simulink model "ResonantEstimator"  (R2019b)
settings: Solver=VariableStepAuto  StartTime=0.0  StopTime=tSim  RelTol=1e-3
values from neighbouring files (symbols this model uses):
  a = 0    [Q4.m]    (also in Sol_Q1.m = 0.1)
  amplitude = 3    [Q4.m]
  deltat = 0.01    [Q4.m]    (also in Sol_Q1.m = 0.001; main3.m; param3.m = 0.001; params2.m = 0.1)
  gamma1 = (2*zeta*wn)/b    (= 4)    [Q4.m]
  gamma2 = (wn^2 - w0^2)/b    (= 7.5)    [Q4.m]
  Gs = tf(b, [1 a])    [Q4.m]    (also in Q5.m = tf([b1 b0], [1 a1 a0]); Sol_Q1.m = tf(num, den); main3.m = tf(num, den); param3.m = tf(b, [1 a1 a0]))
  K1 = (alpha1 - a)/b    (= 1.5)    [Q4.m]    (also in Sol_Q1.m = 5; main3.m = 4; param3.m = 5)
  shift = 2    [Q4.m]
  umax = 8.8    [Q4.m]    (also in Sol_Q1.m = 10000; main3.m = 4.5; param3.m = 999)
  umin = -100    [Q4.m]    (also in Sol_Q1.m = -10000; main3.m = -0.9; param3.m = -999)
  w0 = 1    [Q4.m]
  wn = 4    [Q4.m]    (also in main3.m = 3; param3.m = 3)
  zeta = 1    [Q4.m]    (also in main3.m = 0.707; param3.m = 0.707)
settings Model: Creator=adityaaaap  LastModifiedBy=adityaaaap

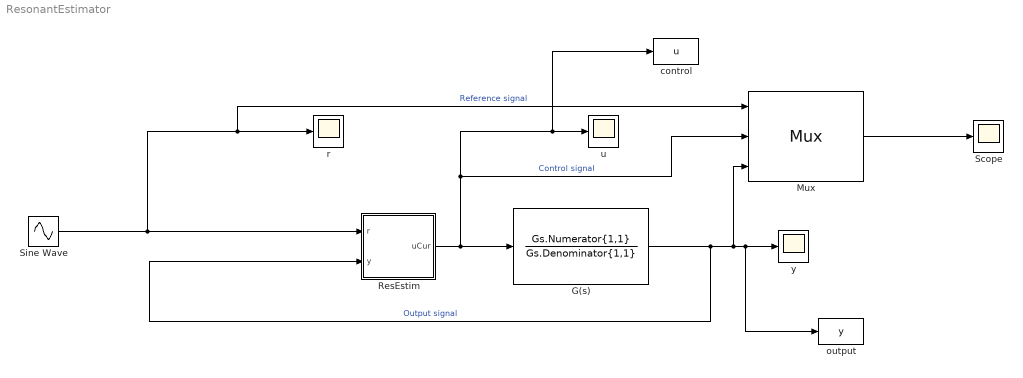
== system ResonantEstimator ==
  G(s) : TransferFcn  Numerator=Gs.Numerator{1,1}  Denominator=Gs.Denominator{1,1}
  Mux : Mux  Inputs=3
      settings: DisplayOption=signals
  "ResEstim " : MATLAB Function  TreatAsAtomicUnit=on
  Scope : Scope
  Sine Wave : Sin  Amplitude=amplitude  Bias=shift  Frequency=w0  SampleTime=deltat
  control : ToWorkspace  VariableName=u
      settings: MaxDataPoints=10000
  output : ToWorkspace  VariableName=y
      settings: MaxDataPoints=10000
  r : Scope
  u : Scope
  y : Scope
  wires:
  Sine Wave/1 -> Mux/1, r/1, "ResEstim "/1(r)  "Reference signal"
  G(s)/1 -> "ResEstim "/2(y), Mux/3, output/1, y/1  "Output signal"
  "ResEstim "/1(uCur) -> Mux/2, control/1, u/1, G(s)/1  "Control signal"
  Mux/1 -> Scope/1

== matlab function ResonantEstimator/ResEstim  ==
  settings: updateMethod=DISCRETE  sampleTime=deltat
  data: r input; uCur output; y input; K1 parameter; gamma1 parameter; gamma2 parameter; zeta parameter; wn parameter; a parameter; w0 parameter; deltat parameter; umin parameter; umax parameter
function uCur =ResEstim(r,y,K1, gamma1, gamma2, zeta, wn, a, w0, deltat, umin, umax)
persistent zhat1
if isempty(zhat1)
zhat1=0;
end
persistent zhat2
if isempty(zhat2)
zhat2=0;
end

cz1=a*gamma1 - 2*zeta*wn*gamma1+gamma2;
cz2=2*zeta*wn;

dhat=zhat1+gamma1*(y-r);
uCur= -K1*(y-r)-dhat;

if (uCur>umax) uCur=umax;end
if (uCur<umin) uCur=umin;end

zhat1=zhat1+deltat*((-cz2*zhat1+zhat2)+cz1*(y-r)-cz2*uCur);
zhat2=zhat2+deltat*(-wn^2*zhat1+(a*gamma2-wn^2*gamma1)*(y-r)-(wn^2-w0^2)*uCur);
